simulink model "spring_damper"  (R2026a)
settings: Solver=ode45  StopTime=50  FixedStep=0.01  MaxStep=0.01
undefined symbols (not defined in the file or in its folder): c, k, m
settings Model: Creator=lenovo  LastModifiedBy=lenovo

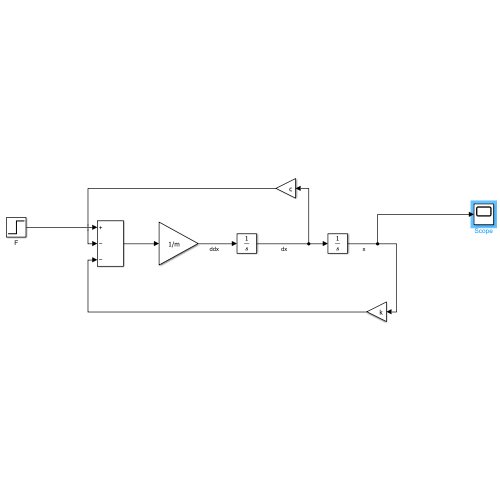
[thumbnail: Simulink's stored preview of the top-level diagram]
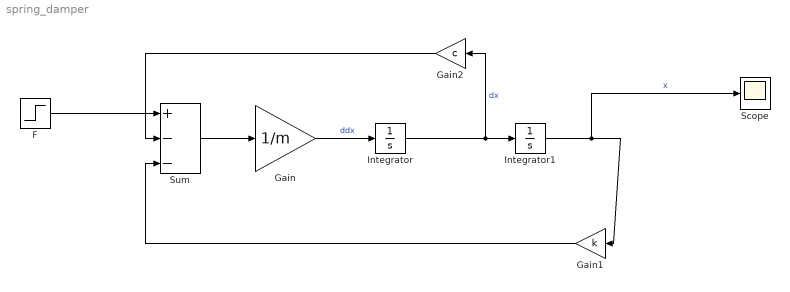
== system spring_damper ==
  F : Step  SampleTime=0
  Gain : Gain  Gain=1/m
  Gain1 : Gain  Gain=k
  Gain2 : Gain  Gain=c
  Integrator : Integrator
  Integrator1 : Integrator
  Scope : Scope
      settings: ActiveDisplayYMinimum=-0.14406538492817428  ActiveDisplayYMaximum=0.27282615580428815
  Sum : Sum  Inputs=+--
  wires:
  Integrator/1 -> Gain2/1, Integrator1/1  "dx"
  Gain/1 -> Integrator/1  "ddx"
  Integrator1/1 -> Scope/1, Gain1/1  "x"
  Sum/1 -> Gain/1
  Gain1/1 -> Sum/3
  Gain2/1 -> Sum/2
  F/1 -> Sum/1
